simulink model "trb"  (R2015a)
settings: Solver=ode45  StartTime=0.0  StopTime=10.0  RelTol=1e-3
libraries: commdigbbndfm2 x2, commchan3 x1, commsink2 x1, commrandsrc2 x1
settings Model: Creator=francisco  LastModifiedBy=francisco

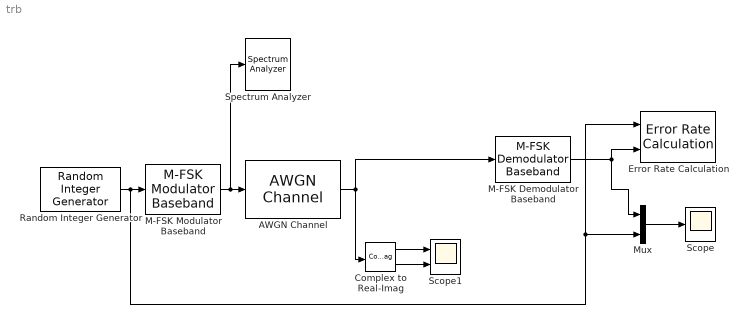
== system trb ==
  AWGN Channel : commchan3/AWGN Channel  InputProcessing=Columns as channels (frame based)  seed=67  noiseMode="Signal to noise ratio  (Eb/No)"  EbNodB=10  EsNodB=10  SNRdB=10  bitsPerSym=1  Ps=1  Tsym=1  variance=1
  Complex to Real-Imag : ComplexToRealImag
  Error Rate Calculation : commsink2/Error Rate Calculation  N=0  st_delay=0  cp_mode=Entire frame  subframe=[]  PMode=Workspace  WsName=ErrorVec  RsMode2=off  stop=off  numErr=100  maxBits=1e6
  M-FSK Demodulator Baseband : commdigbbndfm2/M-FSK Demodulator Baseband  M=2  OutType=Integer  Dec=Gray  freqSep=200  numSamp=17  RateOptions=Enforce single-rate processing  outDataType=double
  M-FSK Modulator Baseband : commdigbbndfm2/M-FSK Modulator Baseband  M=2  InType=Integer  Enc=Gray  freqSep=100  phaseType=Continuous  numSamp=17  RateOptions=Enforce single-rate processing  outDataType=double
  Mux : Mux  Inputs=2
  Random Integer Generator : commrandsrc2/Random Integer Generator  mul=2  seed=37  Ts=0.01  frameBased=off  sampPerFrame=1  orient=off  outDataType=double
  Scope : Scope
      settings: Decimation=100
  Scope1 : Scope  NumInputPorts=2
      settings: YMin=-5~-5  YMax=5~5
  Spectrum Analyzer : SpectrumAnalyzer
  wires:
  Random Integer Generator/1 -> M-FSK Modulator Baseband/1, Error Rate Calculation/1, Mux/2
  M-FSK Demodulator Baseband/1 -> Mux/1, Error Rate Calculation/2
  Mux/1 -> Scope/1
  Complex to Real-Imag/1 -> Scope1/1
  Complex to Real-Imag/2 -> Scope1/2
  AWGN Channel/1 -> M-FSK Demodulator Baseband/1, Complex to Real-Imag/1
  M-FSK Modulator Baseband/1 -> Spectrum Analyzer/1, AWGN Channel/1
